simulink library "xrbsComm_r4"  (Simulink 7.1)
PreLoadFcn:
  | warning('off','MATLAB:mex:deprecatedExtension');xlmeta;com.xilinx.sysgen.util.StrategyUtil.loadAllStrategyNames();
undefined symbols (not defined in the file or in its folder): calc_path_data, gcbh, mfcm_matrix_rom, oct2dec, xlBlockLoadCallback
libraries: xbsIndex_r4 x851, mfcm_block_lib_v1 x5, xrbsComm_r4 x1, mfcm_misc_lib_v1 x1
(part 1 of 8)
settings Model: Tag=SysGenIndex  Creator=singhj  LastModifiedBy=sysgengroup

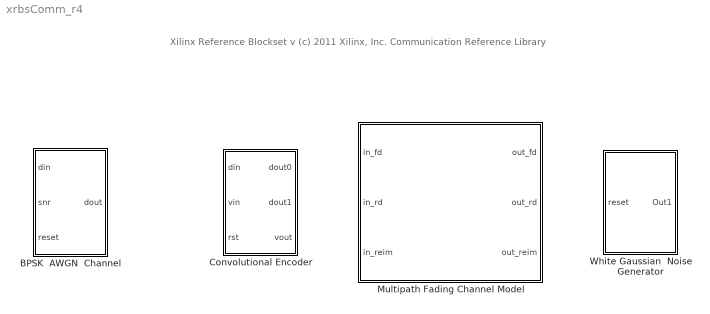
== system xrbsComm_r4 ==
  note: Xilinx Reference Blockset v
      | (c) 2011 Xilinx, Inc.
      |
      | Communication Reference Library
  BPSK  AWGN  Channel : Subsystem  mask(BPSK AWGN Channel){seed=510}
      mask prompts: seed "Decimal Seed Value"
      mask help: Binary Phase Shift Keying Additive White Gaussian Noise Channel. Adds scaled white Gaussian nose to an input signal.
      mask init:
      | [bg,fg] = xlcmap('XBlock',0);
      | iPos = get_param(gcb,'Position');
      | iWidth=iPos(3)-iPos(1); iHeight=iPos(4)-iPos(2);
      | iCx=iWidth/2;
      | iCy=iHeight/2;
      | [logoX, logoY] = xlogo(iPos);
      mask Help: eval('');xlDoc('-book','sysgen','-topic','BPSK_AWGN_Channel');
      mask Display:
      | patch([0 iWidth iWidth 0],[0 0 iHeight iHeight] , bg);
      | patch(logoX,logoY , fg);
      | port_label('input',1,'din');
      | port_label('input',2,'snr');
      | port_label('input',3,'reset');
      | port_label('output',1,'dout');
      | plot([0 0 iWidth iWidth 0], [0 iHeight iHeight 0 0]);
  Convolutional Encoder : Subsystem  mask(Convolutional Encoder Reference Block){K=7, code=[177 133]}
      mask prompts: K "Constraint Length [3 to 9]"; code "Convolutional code array (octal)"
      mask help: The constraint length and convolution code array are controlled by the mask parameters.
      mask init:
      | saved_gcb = gcb;
      | % Because of an issue where I was unable to save state consistently 
      | % when changing parameters and clicking the 'Apply' button, 
      | % I have included the following workaround that determines the number of subsystems.
      | sys_in_convenc = find_system(saved_gcb, 'lookUnderMasks', 'all', 'SearchDepth', 1, 'BlockType', 'SubSystem');
      | subsys_in_convenc = strfind(sys_in_convenc(1:length(sys_in_convenc)), 'Subsystem');
      | found_num_sys = 2;
      | for idx = 1:length(subsys_in_convenc)
      |   if (length(subsys_in_convenc(idx)))
      |     start_of_str = subsys_in_convenc{idx};
      |     length_of_sstr = length('Subsystem');
      |     char_idx_of_interest = start_of_str+length_of_sstr;
      |     
      |     if (char_idx_of_interest <= length(sys_in_convenc{idx}))
      |       char_of_interest = sys_in_convenc{idx}(char_idx_of_interest);
      |       sys_num = str2num(char_of_interest) + 1;
      |       if (sys_num > found_num_sys)
      |         found_num_sys = sys_num;
      |       end
      |     end
      |   end
      | end
      | saved_existing_subsys = found_num_sys;  
      | 
      | 
      | % Code for drawing the System Generator icon.
      | 
      | [bg,fg] = xlcmap('XBlock',0);
      | iPos = get_param(gcb,'Position');
      | iWidth=iPos(3)-iPos(1); iHeight=iPos(4)-iPos(2);
      | iCx=iWidth/2;
      | iCy=iHeight/2;
      | [logoX, logoY] = xlogo(iPos);
      | 
      | 
      | 
      | % Perform error checking on input parameters
      | 
      | err__k_not_int_in_range = false;
      | err__k_not_evaluated = false;
      | if (length(K) ~= 0)
      |   k_int = int32(round(K));
      |   if ((k_int ~= K) | (k_int < 3) | (k_int > 9))
      |     err__k_not_int_in_range = true;
      |   end
      | else
      |   err__k_not_evaluated = true;
      | end
      | err_in_param_k = err__k_not_int_in_range | err__k_not_evaluated;
      | 
      | err__codelen_not_in_range = false;
      | err__code_not_octal = false;
      | err__code_too_large_for_constraint = false;
      | err__code_not_evaluated = false;
      | if (length(code) ~= 0)
      |   code_len = length(code);
      |   if ((code_len < 2) | (code_len > 7))
      |     err__codelen_not_in_range = true;
      |   end
      |   for idx = 1:code_len
      |     try
      |       oct2dec(code(idx));
      |     catch
      |       err__code_not_octal = idx;
      |     end
      |   end
      |   if (~err_in_param_k & (err__code_not_octal == 0))
      |     code_eval_dec = oct2dec(code);
      |     max_code_val = 2^k_int;
      |     err__code_too_large_for_constraint = find(code_eval_dec > max_code_val);
      |     if (length(err__code_too_large_for_constraint) == 0)
      |       err__code_too_large_for_constraint = false;
      |     end
      |   end
      | else
      |   err__code_not_evaluated = true;
      | end
      | err_in_param_code = err__codelen_not_in_range | err__code_not_octal | err__code_too_large_for_constraint | err__code_not_evaluated;
      | 
      | valid_parameters = ~(err_in_param_k | err_in_param_code);
      | 
      | 
      | 
      | % Perform programatic generation of the convolutional encoder if the parameters are valid.
      | 
      | num_subsystems = saved_existing_subsys;
      | if (valid_parameters)
      |   num_subsystems = code_len;
      |   iconStr = '';
      |   if (num_subsystems ~= saved_existing_subsys)  
      |     subsys_proto = [saved_gcb '/Subsystem'];
      |     subsys_proto_dimensions = get_param(subsys_proto, 'Position');
      |     subsys_x = subsys_proto_dimensions(1);
      |     subsys_y = subsys_proto_dimensions(2);
      |     subsys_width = abs(subsys_proto_dimensions(3) - subsys_x);
      |     subsys_height = abs(subsys_proto_dimensions(4) - subsys_y);
      |     distance_between = 1.5*subsys_height;
      |     subsys_x2 = subsys_x+subsys_width;
      | 
      |     subsys_oport = [saved_gcb '/dout0'];
      |     subsys_oport_dimensions = get_param(subsys_oport, 'Position');
      |     subsys_oport_x = subsys_oport_dimensions(1);
      |     subsys_oport_y = subsys_oport_dimensions(2);
      |     subsys_oport_width = abs(subsys_oport_dimensions(3) - subsys_oport_x);
      |     subsys_oport_height = abs(subsys_oport_dimensions(4) - subsys_oport_y);
      |     subsys_oport_x2 = subsys_oport_x+subsys_oport_width;
      |     
      |     subsys_iport_din = 'din/1';
      |     subsys_iport_rst = 'rst/1';
      |     subsys_iport_vin = 'vin/1';
      | 
      |     minimum_subsystems = 2;
      |     if (num_subsystems  < saved_existing_subsys)
      |       for idx = (num_subsystems+1):saved_existing_subsys
      |         subsys_name = ['Subsystem' num2str(idx-1)];
      |         subsys_full_path = [saved_gcb '/' subsys_name];
      | 
      |         oport_name = ['dout' num2str(idx-1)];
      |         oport_full_path = [saved_gcb '/' oport_name];
      |         subsys_output_port = [subsys_name '/1'];
      |         oport_input_port = [oport_name '/1'];
      |         delete_line(saved_gcb, subsys_output_port, oport_input_port);
      |         delete_block(oport_full_path);
      |         
      |         subsys_din_port = [subsys_name '/1'];
      |         subsys_rst_port = [subsys_name '/2'];
      |         subsys_vin_port = [subsys_name '/3'];
      |         delete_line(saved_gcb, subsys_iport_din, subsys_din_port);
      |         delete_line(saved_gcb, subsys_iport_rst, subsys_rst_port);
      |         delete_line(saved_gcb, subsys_iport_vin, subsys_vin_port);
      |         delete_block(subsys_full_path);
      |       end
      |     elseif (num_subsystems > saved_existing_subsys)
      |       for idx = (saved_existing_subsys+1):num_subsystems
      |         subsys_name = ['Subsystem' num2str(idx-1)];
      |         new_subsys = [saved_gcb '/' subsys_name];
      |         y1 = subsys_y+(idx-1)*distance_between;
      |         y2 = subsys_y+subsys_height+(idx-1)*distance_between;
      |         new_position = [subsys_x y1 subsys_x2 y2];
      |         add_block(subsys_proto, new_subsys, 'Position', new_position);
      |         set_param(new_subsys, 'index', num2str(idx));
      |         
      |         oport_name = ['dout' num2str(idx-1)];
      |         new_oport = [saved_gcb '/' oport_name];
      |         y1 = subsys_oport_y+(idx-1)*distance_between;
      |         y2 = subsys_oport_y+subsys_oport_height+(idx-1)*distance_between;
      |         new_position = [subsys_oport_x y1 subsys_oport_x2 y2];
      |         add_block(subsys_oport, new_oport, 'Position', new_position);
      |         
      |         subsys_output_port = [subsys_name '/1'];
      |         oport_input_port = [oport_name '/1'];
      |         add_line(saved_gcb, subsys_output_port, oport_input_port);
      |         
      |         subsys_din_port = [subsys_name '/1'];
      |         subsys_rst_port = [subsys_name '/2'];
      |         subsys_vin_port = [subsys_name '/3'];
      |         add_line(saved_gcb, subsys_iport_din, subsys_din_port, 'autorouting', 'on');
      |         add_line(saved_gcb, subsys_iport_rst, subsys_rst_port, 'autorouting', 'on');
      |         add_line(saved_gcb, subsys_iport_vin, subsys_vin_port, 'autorouting', 'on');
      |       end
      |     end
      |       
      |     % Delete/Re-add the vout block to get the port numbers so that all dout ports
      |     % are grouped together.
      |     vout_block = [saved_gcb '/vout'];
      |     vout_block_pos = get_param(vout_block, 'Position');
      |     delete_block(vout_block);
      |     add_block(subsys_oport, vout_block, 'Position', vout_block_pos);
      |   end
      | else
      |   iconStr = 'ERROR';
      | end
      | 
      | 
      | 
      | % This code generates a vector and cellarray of
      | % port numbers and names respectively to allow
      | % the number of output ports to be changed.
      | % (Their is no way to change the icon Drawing
      | % Code dynamically--i.e. it doesn't allow
      | % loop constructs, hence all the add ports.)
      | 
      | num_dout_ports = num_subsystems;
      | max_out_ports = 8;
      | out_port_nums = [];
      | out_port_names = {};
      | for idx = 1:max_out_ports
      |   if (idx <= num_dout_ports)
      |     out_port_nums = [out_port_nums idx];
      |     out_port_names = [out_port_names {['dout' num2str(idx)]}];
      |   else
      |     out_port_nums = [out_port_nums (num_dout_ports+1)];
      |     out_port_names = [out_port_names {'vout'}];
      |   end;
      | end
      | 
      | 
      | 
      | % Present any errors or warnings to users
      | 
      | if (err__k_not_evaluated)
      |   errordlg([saved_gcb ': Constraint length could not be evaluated.']);
      | elseif (err__k_not_int_in_range)
      |   errordlg([saved_gcb ': Constraint length is set to ' num2str(K) ', but must be an integer between 3 and 9, inclusive.']);
      | elseif(err__code_not_evaluated)
      |   errordlg([saved_gcb ': The convolution code array could not be evaluated.']);
      | elseif(err__code_too_large_for_constraint)
      |   errordlg([saved_gcb ': The convolution code array value(s) at position(s): ' num2str(err__code_too_large_for_constraint) ', are too large for the constraint length, ' num2str(K) '.']);
      | elseif(err__code_not_octal)
      |   errordlg([saved_gcb ': The convolution code array must contain octal numbers only (i.e. only numbers containing the digits 0-7).  The value at position ' num2str(err__code_not_octal) ' is not an octal value.']);
      | elseif(err__codelen_not_in_range)
      |   errordlg([saved_gcb ': The length of the convolution code array must be between 2 and 7, inclusive.']);
      | end
      settings: CopyFcn=set_param(gcb, 'MaskSelfModifiable', 'on', 'LinkStatus', 'none');
      mask Help: eval('');xlDoc('-book','sysgen','-topic','Convolutional_Encoder');
      mask Display:
      | patch([0 iWidth iWidth 0],[0 0 iHeight iHeight] , bg);
      | patch(logoX,logoY , fg);
      | port_label('input',1,'din');
      | port_label('input',2,'vin');
      | port_label('input',3,'rst');
      | port_label('output', out_port_nums(1), char(out_port_names{1}));
      | port_label('output', out_port_nums(2), char(out_port_names{2}));
      | port_label('output', out_port_nums(3), char(out_port_names{3}));
      | port_label('output', out_port_nums(4), char(out_port_names{4}));
      | port_label('output', out_port_nums(5), char(out_port_names{5}));
      | port_label('output', out_port_nums(6), char(out_port_names{6}));
      | port_label('output', out_port_nums(7), char(out_port_names{7}));
      | port_label('output', out_port_nums(8), char(out_port_names{8}));
      | disp(iconStr, 'texmode', 'on');
      | plot([0 0 iWidth iWidth 0], [0 iHeight iHeight 0 0]);
  Multipath Fading Channel Model : Subsystem  LoadFcn=xlBlockLoadCallback(gcbh);  mask(Multipath Fading Channel Model Block){infoedit=Multipath Fading Channel Model., DELAY=[0], GAIN=[1], RT=eye(4,4), RR=eye(4,4), SPEC_DATA=calc_path_data(zeros(4,4,1)+2,ones(4,4,1)), RATE=64, DATAPATH_WIDTH=18, TX_BINPT=17, FADE_BINPT=15, RX_BINPT=15, MAT_BINPT=17, SEED='461AF8228C9F8C92', has_advanced_control=0, sggui_pos=-1,-1,-1,-1, block_type=mfcm, block_version=, sg_icon_stat=180,156,-1,-1,white,blue,0,07734,right,,[ ],[ ], sg_mask_display=|, sg_list_contents=, sg_blockgui_xml=}
      mask sg_mask_display=|
      | fprintf('','COMMENT: begin icon graphics');
      | patch([0 180 180 0 0 ],[0 0 156 156 0 ],[0.77 0.82 0.91 ]);
      | plot([0 180 180 0 0 ],[0 0 156 156 0 ]);
      | patch([41.05 72.84 94.84 116.84 138.84 94.84 63.05 41.05 ],[102.42 102.42 124.42 102.42 124.42 124.42 124.42 102.42 ],[1 1 1 ]);
      | patch([63.05 94.84 72.84 41.05 63.05 ],[80.42 80.42 102.42 102.42 80.42 ],[0.931 0.946 0.973 ]);
      | patch([41.05 72.84 94.84 63.05 41.05 ],[58.42 58.42 80.42 80.42 58.42 ],[1 1 1 ]);
      | patch([63.05 138.84 116.84 94.84 72.84 41.05 63.05 ],[36.42 36.42 58.42 36.42 58.42 58.42 36.42 ],[0.931 0.946 0.973 ]);
      | fprintf('','COMMENT: end icon graphics');
      | fprintf('','COMMENT: begin icon text');
      | fprintf('','COMMENT: end icon text');disp(sprintf('Tx=%d Rx=%d\nPATHS=%d',size(RT,1),size(RR,1),length(GAIN)),'texmode','on');
      mask prompts: infoedit ""; DELAY "Path Delay Vector"; GAIN "Path Gain Vector"; RT "Transmit Array Spatial Covariance Matrices"; RR "Receive Array Spatial Covariance Matrices"; SPEC_DATA "Spectrum Data"; DATAPATH_WIDTH "Datapath Width in Bits"; TX_BINPT "Transmit Multiply Binary Point"; FADE_BINPT "Fading Multiply Binary Point"; RX_BINPT "Receive Multiply Binary Point"; MAT_BINPT "Covariance Matrix Binary Point"; SEED "Random Seed"; has_advanced_control ""; sggui_pos ""; block_type ""; block_version ""; sg_icon_stat ""; sg_mask_display ""; sg_list_contents ""; sg_blockgui_xml ""
      mask help: Multipath Fading Channel Model.
      mask init:
      | try
      |   tmp_gcb = gcb;
      |   tmp_gcbh = gcbh;
      |   if (strcmp('SysGenIndex',get_param(bdroot(tmp_gcbh),'tag')) && ~isempty(regexp(bdroot(tmp_gcb), '^xbs', 'once')))
      |     return;
      |   end;
      |   xlMungeMaskParams;
      | 
      |   block_type='mfcm';
      | 
      |   serialized_declarations = '{''block_type''=>''String''}';
      |   ptable_ = xlblockprep(get_param(tmp_gcb, 'MaskWSVariables'));
      |   try
      |     xlBlockMoveCallback(tmp_gcbh);
      |   catch 
      |      clear global xl_updateicon_recursion_guard;
      |   end;
      | catch
      |   global dbgsysgen;
      |   if(~isempty(dbgsysgen) && dbgsysgen)
      |     e = regexprep(lasterr, '\n', '\nError: ');
      |     disp(['Error: While running MaskInit code on block ' tmp_gcb ': ' e]);
      |     error(e);
      |   end
      | end
      settings: CopyFcn=xlBlockMoveCallback(gcbh);  DeleteFcn=xlDestroyGui(gcbh);  ModelCloseFcn=xlDestroyGui(gcbh);  PreSaveFcn=xlBlockPreSaveCallback(gcbh);  PostSaveFcn=xlBlockPostSaveCallback(gcbh);  DestroyFcn=xlDestroyGui(gcbh);  OpenFcn=xlOpenGui(gcbh, 'mfcm_gui.xml', -1, -1)  CloseFcn=xlDestroyGui(gcbh);  MoveFcn=xlBlockMoveCallback(gcbh);
      mask Help: eval('');xlDoc('-book','sysgen','-topic','Multipath_Fading_Channel_Model');
      mask Display:
      | fprintf('','COMMENT: begin icon graphics');
      | patch([0 180 180 0 0 ],[0 0 156 156 0 ],[0.77 0.82 0.91 ]);
      | plot([0 180 180 0 0 ],[0 0 156 156 0 ]);
      | patch([41.05 72.84 94.84 116.84 138.84 94.84 63.05 41.05 ],[102.42 102.42 124.42 102.42 124.42 124.42 124.42 102.42 ],[1 1 1 ]);
      | patch([63.05 94.84 72.84 41.05 63.05 ],[80.42 80.42 102.42 102.42 80.42 ],[0.931 0.946 0.973 ]);
      | patch([41.05 72.84 94.84 63.05 41.05 ],[58.42 58.42 80.42 80.42 58.42 ],[1 1 1 ]);
      | patch([63.05 138.84 116.84 94.84 72.84 41.05 63.05 ],[36.42 36.42 58.42 36.42 58.42 58.42 36.42 ],[0.931 0.946 0.973 ]);
      | fprintf('','COMMENT: end icon graphics');
      | fprintf('','COMMENT: begin icon text');
      | fprintf('','COMMENT: end icon text');disp(sprintf('Tx=%d Rx=%d\nPATHS=%d',size(RT,1),size(RR,1),length(GAIN)),'texmode','on');
  White Gaussian  Noise Generator : Subsystem  mask(White Gaussian Noise Generator){seed=512}
      mask help: White Gaussian Noise Generator. Generates white Gaussian noise using a combination of the Box-Muller algorithm and the central limit theorem.
      mask init:
      | old_seed = rand('seed');
      | rand('seed',seed);
      | init1 = [dec2hex(floor(rand*16)) dec2hex(floor(rand*16)) dec2hex(floor(rand*16)) ...
      | 		dec2hex(floor(rand*16)) dec2hex(floor(rand*16)) dec2hex(floor(rand*16)) ...
      | 		dec2hex(floor(rand*16)) dec2hex(floor(rand*16)) dec2hex(floor(rand*16)) ...
      | 		dec2hex(floor(rand*16)) dec2hex(floor(rand*16)) dec2hex(floor(rand*16))];
      | seed1 = hex2dec(init1);
      | init2 = [dec2hex(floor(rand*16)) dec2hex(floor(rand*16)) dec2hex(floor(rand*16)) ...
      | 		dec2hex(floor(rand*16)) dec2hex(floor(rand*16)) dec2hex(floor(rand*16)) ...
      | 		dec2hex(floor(rand*16)) dec2hex(floor(rand*16)) dec2hex(floor(rand*16)) ...
      | 		dec2hex(floor(rand*16)) dec2hex(floor(rand*16)) dec2hex(floor(rand*16))];
      | seed2 = hex2dec(init2);
      | init3 = [dec2hex(floor(rand*16)) dec2hex(floor(rand*16)) dec2hex(floor(rand*16)) ...
      | 		dec2hex(floor(rand*16)) dec2hex(floor(rand*16)) dec2hex(floor(rand*16)) ...
      | 		dec2hex(floor(rand*16)) dec2hex(floor(rand*16)) dec2hex(floor(rand*16)) ...
      | 		dec2hex(floor(rand*16)) dec2hex(floor(rand*16)) dec2hex(floor(rand*16))];
      | seed3 = hex2dec(init3);
      | init4 = [dec2hex(floor(rand*16)) dec2hex(floor(rand*16)) dec2hex(floor(rand*16)) ...
      | 		dec2hex(floor(rand*16)) dec2hex(floor(rand*16)) dec2hex(floor(rand*16)) ...
      | 		dec2hex(floor(rand*16)) dec2hex(floor(rand*16)) dec2hex(floor(rand*16)) ...
      | 		dec2hex(floor(rand*16)) dec2hex(floor(rand*16)) dec2hex(floor(rand*16))];
      | seed4 = hex2dec(init4);
      | rand('seed',old_seed);
      | 
      | 
      | [bg,fg] = xlcmap('XBlock',0);
      | iPos = get_param(gcb,'Position');
      | iWidth=iPos(3)-iPos(1); iHeight=iPos(4)-iPos(2);
      | iCx=iWidth/2;
      | iCy=iHeight/2;
      | [logoX, logoY] = xlogo(iPos);
      mask Help: eval('');xlDoc('-book','sysgen','-topic','White_Gaussian_Noise_Generator');
      mask Display:
      | patch([0 iWidth iWidth 0],[0 0 iHeight iHeight] , bg);
      | patch(logoX,logoY , fg);
      | port_label('input',1,'reset');
      | port_label('output',1,'noise');
      | plot([0 0 iWidth iWidth 0], [0 iHeight iHeight 0 0]);

== system xrbsComm_r4/BPSK  AWGN  Channel ==
  note: The WGNG block generates a probability density function (PDF) that is Gaussian to within .2% for
      | 4.8 standard deviations from the mean.  The PDF is scaled based on the value of the signal to noise
      | ratio to achieve the desired noise variance.  The SNR input is defined as (Eb/No) in dB for uncoded BPSK
      | with unit symbol energy (Es = 1).  If the SNR input is of type UFix8_4, the valid range is from 0.0 to 15.9375
      | in steps of 0.0625dB.  To use the AWGN in a system with coding and/or to use the core with different
      | modulation formats, it is necessary to adjust the SNR value to accommodate the difference in spectral
      | efficiency.  If we have BPSK modulation with rate 1/2 coding and keep Es = 1and No constant, then Eb = 2
      | and Eb/No = SNR + 3 dB.  If we have uncoded QPSK modulation with I = +/-1 and Q = +/-1 and add
      | independent noise sequences, then each channel looks like and independent BPSK channel and the
      | Eb/No = SNR.  If we then add rate 1/2 coding to the QPSK case, we have Eb/No = SNR + 3 dB.
      |
      | For more information see:
      |
      | [1] A. Ghazel, E. Boutillon, J. L. Danger, G. Gulak and H. Laamari, "Design and Performance Analysis of a
      | High Speed AWGN Communication Channel Emulator" IEEE PACRIM Conference, Victoria, B. C., Aug.
      | 2001.
      | [2] Xilinx Data Sheet: Additive White Gaussian Noise (AWGN) Core v1.0, Xilinx, Inc. October 2002
  din : Inport  OutDataType=sfix(16)  OutScaling=2^0
  snr : Inport  Port=2  OutDataType=sfix(16)  OutScaling=2^0
  reset : Inport  Port=3  OutDataType=sfix(16)  OutScaling=2^0
  AddSub : xbsIndex_r4/AddSub  mode=Addition  use_carryin=off  use_carryout=off  en=off  latency=1  precision=Full  arith_type=Unsigned  n_bits=8  bin_pt=2  quantization=Truncate  overflow=Wrap  dbl_ovrd=off  use_behavioral_HDL=on  pipelined=off  use_rpm=off  block_type=addsub
      settings: xl_area=[0, 0, 0, 0, 0, 0, 0]  block_version=VER_STRING_GOES_HERE
  Constant1 : xbsIndex_r4/Constant  arith_type=Signed (2's comp)  const=1  n_bits=2  bin_pt=0  explicit_period=off  period=1  equ=P=C  opselect=C  inp2=PCIN>>17  opr=+  inp1=P  carry=CIN  dbl_ovrd=off  block_type=constant
      settings: block_version=VER_STRING_GOES_HERE
  Constant2 : xbsIndex_r4/Constant  arith_type=Signed (2's comp)  const=-1  n_bits=2  bin_pt=0  explicit_period=off  period=1  equ=P=C  opselect=C  inp2=PCIN>>17  opr=+  inp1=P  carry=CIN  dbl_ovrd=off  block_type=constant
      settings: block_version=VER_STRING_GOES_HERE
  Convert : xbsIndex_r4/Convert  arith_type="Signed  (2's comp)"  n_bits=16  bin_pt=11  quantization="Round  (unbiased: +/- Inf)"  overflow=Wrap  latency=2  dbl_ovrd=off  pipeline=off  block_type=convert
      settings: infoedit=The input is presented at the output after quantization and overflow effects.<P><P>Hardware notes: Additional hardware is used when rounding or saturation is selected and output width is less than the input width.  xl_area=[0, 0, 0, 0, 0, 0, 0]  block_version=VER_STRING_GOES_HERE
  Delay : xbsIndex_r4/Delay  en=off  latency=14  dbl_ovrd=off  reg_retiming=off  block_type=delay
      settings: infoedit="Delay line having  configurable length.<P><P>Hardware notes: A delay line is a chain, each link of which is an SRL16 followed by a flip-flop. If register retiming is enabled, the delay line is a chain of flip-flops."  xl_area=[0, 0, 0, 0, 0, 0, 0]  block_version=VER_STRING_GOES_HERE
  Input  Conversion : Subsystem
  Mult : xbsIndex_r4/Mult  precision=Full  arith_type="Signed  (2's comp)"  n_bits=8  bin_pt=2  quantization=Truncate  overflow=Wrap  en=off  latency=2  dbl_ovrd=off  use_behavioral_HDL=off  use_embedded=on  pipeline=off  use_rpm=off  placement_style=Rectangular shape  block_type=mult
      settings: infoedit=Multiplies two values.<P><P>Hardware notes: To use the internal pipeline stage of the dedicated multiplier you must select 'Pipeline to Greatest Extent Possible'.  xl_area=[0, 0, 0, 0, 0, 0, 0]  block_version=VER_STRING_GOES_HERE
  Mux : xbsIndex_r4/Mux  inputs=2  en=off  latency=0  precision=Full  arith_type="Signed  (2's comp)"  n_bits=8  bin_pt=2  quantization=Truncate  overflow=Wrap  dbl_ovrd=off  block_type=mux
      settings: xl_area=[0, 0, 0, 0, 0, 0, 0]  block_version=VER_STRING_GOES_HERE
  ROM : xbsIndex_r4/ROM  depth=256  initVector=((2*10.^(0.1*(([0:255]/10) - 0.6*floor([0:255]/16) ))).^(-0.5))*1.0023  distributed_mem=Block RAM  rst=off  init_reg=0  en=off  latency=1  arith_type=Unsigned  n_bits=15  bin_pt=15  dbl_ovrd=off  use_rpm=off  block_type=sprom
      settings: xl_area=[0, 0, 0, 0, 0, 0, 0]  block_version=VER_STRING_GOES_HERE
  White Gaussian  Noise Generator : xrbsComm_r4/White Gaussian  Noise Generator  seed=seed
  dout : Outport  OutDataType=sfix(16)  OutScaling=2^0
  wires:
  reset/1 -> White Gaussian  Noise Generator/1
  Delay/1 -> AddSub/1
  Convert/1 -> AddSub/2
  White Gaussian  Noise Generator/1 -> Mult/2
  din/1 -> Mux/1
  snr/1 -> Input  Conversion/1(" ")
  Mult/1 -> Convert/1
  ROM/1 -> Mult/1
  AddSub/1 -> dout/1
  Input  Conversion/1(conv) -> ROM/1
  Constant1/1 -> Mux/2
  Constant2/1 -> Mux/3
  Mux/1 -> Delay/1

== system xrbsComm_r4/Convolutional Encoder ==
  din : Inport  OutDataType=sfix(16)  OutScaling=2^0
  vin : Inport  Port=2  OutDataType=sfix(16)  OutScaling=2^0
  rst : Inport  Port=3  OutDataType=sfix(16)  OutScaling=2^0
  More Info : Subsystem
      mask Display: disp('Double click\n for\n more information.')
  Subsystem : Subsystem  mask{index=1}
  Subsystem1 : Subsystem  mask{index=2}
  Valid Out Logic : Subsystem
  dout0 : Outport  OutDataType=sfix(16)  OutScaling=2^0
  dout1 : Outport  Port=2  OutDataType=sfix(16)  OutScaling=2^0
  vout : Outport  Port=3  OutDataType=sfix(16)  OutScaling=2^0
  wires:
  rst/1 -> Valid Out Logic/2(rst), Subsystem/2(rst), Subsystem1/2(rst)
  din/1 -> Subsystem1/1(din), Subsystem/1(din)
  Valid Out Logic/1(vout) -> vout/1
  Subsystem/1(dout) -> dout0/1
  Subsystem1/1(dout) -> dout1/1
  vin/1 -> Valid Out Logic/1(vin), Subsystem1/3(vin), Subsystem/3(vin)

== system xrbsComm_r4/Multipath Fading Channel Model ==
  in_fd : Inport  OutDataType=sfix(16)  OutScaling=2^0
  in_rd : Inport  Port=2  OutDataType=sfix(16)  OutScaling=2^0
  in_reim : Inport  Port=3  OutDataType=sfix(16)  OutScaling=2^0
  assert[in_fd] : mfcm_misc_lib_v1/assert_width_period  SystemSampleTime=-1  MIN_WIDTH=1  MAX_WIDTH=1  MIN_PERIOD=2*length(GAIN)*max(max(size(RT,1),size(RR,1))^2,size(RT,1)*size(RR,1)*ceil(64/RATE))  MAX_PERIOD=0
  input delay line : mfcm_block_lib_v1/input delay line  SystemSampleTime=-1  MT=size(RT,1)  DELAY=DELAY
  matrix ops : Subsystem  AncestorBlock=mfcm_lib_v1/Multipath Fading Channel Model/matrix ops  mask{MATS=mfcm_matrix_rom(RT,GAIN,RR)}
      mask prompts: MATS "Matrix ROM data"
  out_fd : Outport  OutDataType=sfix(16)  OutScaling=2^0
  out_rd : Outport  Port=2  OutDataType=sfix(16)  OutScaling=2^0
  out_reim : Outport  Port=3  OutDataType=sfix(16)  OutScaling=2^0
  wires:
  matrix ops/3(out_reim) -> out_reim/1
  matrix ops/2(out_rd) -> out_rd/1
  matrix ops/1(out_fd) -> out_fd/1
  in_reim/1 -> input delay line/3
  in_rd/1 -> input delay line/2
  in_fd/1 -> assert[in_fd]/1, input delay line/1
  input delay line/3 -> matrix ops/3(in_reim)
  input delay line/2 -> matrix ops/2(in_rd)
  input delay line/1 -> matrix ops/1(in_fd)

== system xrbsComm_r4/White Gaussian  Noise Generator ==
  note: The WGNG generates white Gaussian noise using a combination of the Box-Muller algorithm and the Central Limit Theorem
      | following the general approach described in [1].   The Box-Muller algorithm generates a unit normal random variable via a
      | transformation of two independent random variables that are uniformly distributed over [0,1].  This is accomplished by storing
      | Box-Muller function values in ROMs and addressing them with uniform random variables.  The uniform random variables are
      | produced by multiple-bit leap-forward LFSRs.  A standard LFSR generates one output per clock cycle.  K-bit leap-forward LFSRs
      | are able to generate k outputs in a single cycle.  For example, a 4-bit leap-forward LFSR outputs a discrete uniform random
      | variable between 0 and 15.  A portion of the 48-bit block parameter seed initializes each LFSR allowing customization.  The
      | outputs of four parallel Box-Muller subsystems are averaged to obtain a probability density function (PDF) that is Gaussian.
      | The overall latency of the WGNG is 10 clock cycles.  The output port noise is a 12 bit signed number with 7 bits after the binary
      | point.
      |
      | [1] A. Ghazel, E. Boutillon, J. L. Danger, G. Gulak and H. Laamari, "Design and Performance Analysis of a
      | High Speed AWGN Communication Channel Emulator" IEEE PACRIM Conference, Victoria, B. C., Aug. 2001.
  " reset" : Inport  OutDataType=sfix(16)  OutScaling=2^0
  AddSub : xbsIndex_r4/AddSub  mode=Addition  use_carryin=off  use_carryout=off  en=off  latency=1  precision=Full  arith_type=Unsigned  n_bits=8  bin_pt=2  quantization=Truncate  overflow=Wrap  dbl_ovrd=off  use_behavioral_HDL=on  pipelined=off  use_rpm=off  block_type=addsub
      settings: xl_area=[0, 0, 0, 0, 0, 0, 0]  block_version=VER_STRING_GOES_HERE
  AddSub1 : xbsIndex_r4/AddSub  mode=Addition  use_carryin=off  use_carryout=off  en=off  latency=1  precision=Full  arith_type=Unsigned  n_bits=8  bin_pt=2  quantization=Truncate  overflow=Wrap  dbl_ovrd=off  use_behavioral_HDL=on  pipelined=off  use_rpm=off  block_type=addsub
      settings: xl_area=[0, 0, 0, 0, 0, 0, 0]  block_version=VER_STRING_GOES_HERE
  AddSub2 : xbsIndex_r4/AddSub  mode=Addition  use_carryin=off  use_carryout=off  en=off  latency=1  precision=Full  arith_type=Unsigned  n_bits=8  bin_pt=2  quantization=Truncate  overflow=Wrap  dbl_ovrd=off  use_behavioral_HDL=on  pipelined=off  use_rpm=off  block_type=addsub
      settings: xl_area=[0, 0, 0, 0, 0, 0, 0]  block_version=VER_STRING_GOES_HERE
  Box-Muller1 : Subsystem  mask(Box-Muller){f_init1=bitget(seed1, 17:-1:1), f_init2=bitget(seed1, 25:-1:1), f_init3=bitget(seed1, 29:-1:1), f_init4=bitget(seed1, 31:-1:1), f_init5=bitget(seed1, 41:-1:1), g_init=bitget(seed1, 47:-1:1)}
      mask prompts: f_init1 "f_init1(17:1)"; f_init2 "f_init2(25:1)"; f_init3 "f_init3(29:1)"; f_init4 "f_init4(31:1)"; f_init5 "f_init5(41:1)"; g_init "g_init(47:1)"
  Box-Muller2 : Subsystem  mask(Box-Muller){f_init1=bitget(seed2, 17:-1:1), f_init2=bitget(seed2, 25:-1:1), f_init3=bitget(seed2, 29:-1:1), f_init4=bitget(seed2, 31:-1:1), f_init5=bitget(seed2, 41:-1:1), g_init=bitget(seed2, 47:-1:1)}
      mask prompts: f_init1 "f_init1(17:1)"; f_init2 "f_init2(25:1)"; f_init3 "f_init3(29:1)"; f_init4 "f_init4(31:1)"; f_init5 "f_init5(41:1)"; g_init "g_init(47:1)"
  Box-Muller3 : Subsystem  mask(Box-Muller){f_init1=bitget(seed3, 17:-1:1), f_init2=bitget(seed3, 25:-1:1), f_init3=bitget(seed3, 29:-1:1), f_init4=bitget(seed3, 31:-1:1), f_init5=bitget(seed3, 41:-1:1), g_init=bitget(seed3,47:-1:1)}
      mask prompts: f_init1 "f_init1(17:1)"; f_init2 "f_init2(25:1)"; f_init3 "f_init3(29:1)"; f_init4 "f_init4(31:1)"; f_init5 "f_init5(41:1)"; g_init "g_init(47:1)"
  Box-Muller4 : Subsystem  mask(Box-Muller){f_init1=bitget(seed4, 17:-1:1), f_init2=bitget(seed4, 25:-1:1), f_init3=bitget(seed4, 29:-1:1), f_init4=bitget(seed4, 31:-1:1), f_init5=bitget(seed4, 41:-1:1), g_init=bitget(seed4, 47:-1:1)}
      mask prompts: f_init1 "f_init1(17:1)"; f_init2 "f_init2(25:1)"; f_init3 "f_init3(29:1)"; f_init4 "f_init4(31:1)"; f_init5 "f_init5(41:1)"; g_init "g_init(47:1)"
  Reinterpret : xbsIndex_r4/Reinterpret  force_arith_type=off  arith_type=Unsigned  force_bin_pt=on  bin_pt=7  block_type=cast
      settings: infoedit="Changes type of samples without altering their binary representation.<P><P>Hardware notes: In hardware this block costs nothing.<P><P>Example:  Suppose the input is 6 bits wide, signed, with 2 fractional bits, and the output is forced to unsigned with 0 fractional bits.  Then an input of -2.0 (1110.00 in binary 2's complement) becomes an output of 56 (111000 in binary)."  block_version=VER_STRING_GOES_HERE
  Out1 : Outport  OutDataType=sfix(16)  OutScaling=2^0
  wires:
  " reset"/1 -> Box-Muller3/1(reset), Box-Muller4/1(reset), Box-Muller2/1(reset), Box-Muller1/1(" reset")
  Reinterpret/1 -> Out1/1
  Box-Muller4/1(bm) -> AddSub1/2
  Box-Muller3/1(bm) -> AddSub1/1
  Box-Muller2/1(bm) -> AddSub/2
  Box-Muller1/1(bm) -> AddSub/1
  AddSub2/1 -> Reinterpret/1
  AddSub1/1 -> AddSub2/2
  AddSub/1 -> AddSub2/1

== system xrbsComm_r4/BPSK  AWGN  Channel/Input  Conversion ==
  " " : Inport  OutDataType=sfix(16)  OutScaling=2^0
  AddSub1 : xbsIndex_r4/AddSub  mode=Addition  use_carryin=off  use_carryout=off  en=off  latency=0  precision=User Defined  arith_type=Unsigned  n_bits=8  bin_pt=0  quantization=Truncate  overflow=Wrap  dbl_ovrd=off  use_behavioral_HDL=on  pipelined=off  use_rpm=off  block_type=addsub
      settings: xl_area=[0, 0, 0, 0, 0, 0, 0]  block_version=VER_STRING_GOES_HERE
  CMult : xbsIndex_r4/CMult  const=16  const_n_bits=5  const_bin_pt=0  en=off  latency=0  precision=Full  arith_type="Signed  (2's comp)"  n_bits=8  bin_pt=6  quantization="Round  (unbiased: +/- Inf)"  overflow=Wrap  dbl_ovrd=off  use_behavioral_HDL=off  mem_type=Distributed RAM  placement_style=Rectangular Shape  pipeline=off  use_rpm=off  block_type=cmult
      settings: xl_area=[0, 0, 0, 0, 0, 0, 0]  block_version=VER_STRING_GOES_HERE
  CMult1 : xbsIndex_r4/CMult  const=10  const_n_bits=4  const_bin_pt=0  en=off  latency=0  precision=Full  arith_type="Signed  (2's comp)"  n_bits=8  bin_pt=6  quantization="Round  (unbiased: +/- Inf)"  overflow=Wrap  dbl_ovrd=off  use_behavioral_HDL=off  mem_type=Distributed RAM  placement_style=Rectangular Shape  pipeline=off  use_rpm=off  block_type=cmult
      settings: xl_area=[0, 0, 0, 0, 0, 0, 0]  block_version=VER_STRING_GOES_HERE
  Shift : xbsIndex_r4/Shift  shift_dir=Right  shift_bits=4  en=off  latency=0  precision=User Defined  arith_type=Unsigned  n_bits=4  bin_pt=0  quantization=Truncate  overflow=Wrap  dbl_ovrd=off  block_type=shift
      settings: xl_area=[0, 0, 0, 0, 0, 0, 0]  block_version=VER_STRING_GOES_HERE
  Slice : xbsIndex_r4/Slice  nbits=4  boolean_output=off  mode=Upper Bit Location + Width  bit1=0  base1=MSB of Input  bit0=0  base0=LSB of Input  dbl_ovrd=off  block_type=slice
      settings: infoedit="Extracts a given range of bits from each input sample and presents it at the output.  The output type is ordinarily unsigned with binary point at zero, but can be Boolean when the slice is one bit wide.<P><P>Hardware notes: In hardware this block costs nothing."  block_version=VER_STRING_GOES_HERE
  Slice1 : xbsIndex_r4/Slice  nbits=4  boolean_output=off  mode=Lower Bit Location + Width  bit1=0  base1=MSB of Input  bit0=0  base0=LSB of Input  dbl_ovrd=off  block_type=slice
      settings: infoedit="Extracts a given range of bits from each input sample and presents it at the output.  The output type is ordinarily unsigned with binary point at zero, but can be Boolean when the slice is one bit wide.<P><P>Hardware notes: In hardware this block costs nothing."  block_version=VER_STRING_GOES_HERE
  conv : Outport  OutDataType=sfix(16)  OutScaling=2^0
  wires:
  Slice/1 -> CMult/1
  Slice1/1 -> CMult1/1
  AddSub1/1 -> conv/1
  CMult/1 -> AddSub1/1
  " "/1 -> Slice/1, Slice1/1
  CMult1/1 -> Shift/1
  Shift/1 -> AddSub1/2

== system xrbsComm_r4/Convolutional Encoder/More Info ==
  note: For example, the octal convolutional codes
      | are shifted and bits from those are used to
      | drive the inputs of the AND gates at left.
      | Any AND gate with a '1' on one input will
      | collapse to a wire.  Any AND gate with a '0'
      | on one input will get pruned away, along
      | with all logic driving the other input of the
      | AND gate.
  note: When the AND gates get pruned, some of the
      | XOR gates have a constant 0 input.  These
      | will get pruned as well.
  note: The 9-bit shift register has been replicated twice
      | simply to make the drawing cleaner.  The
      | synthesizer will collapse these three registers
      | into a single 9-bit shifter.
  note: This block works using a form of parameterizable
      | mux-based collapsing.  This is a method in which
      | constants drive logic blocks.  All logic driven by
      | a constant will be optimized away by the
      | sythesizer.
  note: Parameterizable Mux-Based Collapsing

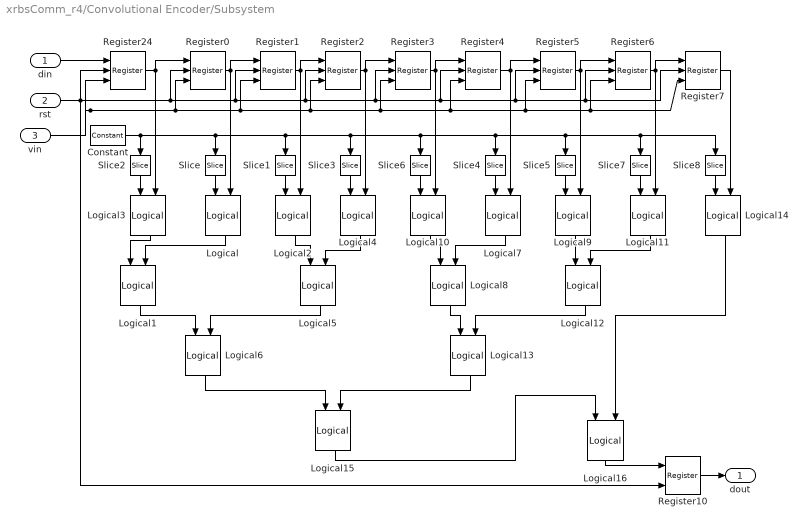
== system xrbsComm_r4/Convolutional Encoder/Subsystem ==
  din : Inport  OutDataType=sfix(16)  OutScaling=2^0
  rst : Inport  Port=2  OutDataType=sfix(16)  OutScaling=2^0
  vin : Inport  Port=3  OutDataType=sfix(16)  OutScaling=2^0
  Constant : xbsIndex_r4/Constant  arith_type=Unsigned  const=oct2dec(code(index))*2^(9-K)  n_bits=9  bin_pt=0  explicit_period=off  period=1  equ=P=C  opselect=C  inp2=PCIN>>17  opr=+  inp1=P  carry=CIN  dbl_ovrd=off  block_type=constant
      settings: block_version=VER_STRING_GOES_HERE
  Logical{,2..4,7,9..11,14} (9 alike) : xbsIndex_r4/Logical  Orientation=down  logical_function=AND  inputs=2  en=off  latency=0  precision=Full  arith_type=Unsigned  n_bits=16  bin_pt=0  align_bp=on  dbl_ovrd=off  block_type=logical
      settings: block_version=VER_STRING_GOES_HERE
  Logical{1,5..6,8,12..13,15..16} (8 alike) : xbsIndex_r4/Logical  Orientation=down  logical_function=XOR  inputs=2  en=off  latency=0  precision=Full  arith_type=Unsigned  n_bits=16  bin_pt=0  align_bp=on  dbl_ovrd=off  block_type=logical
      settings: block_version=VER_STRING_GOES_HERE
  Register{0..7,24} (9 alike) : xbsIndex_r4/Register  init=0  rst=on  en=on  dbl_ovrd=off  block_type=register
      settings: block_version=VER_STRING_GOES_HERE
  Register10 : xbsIndex_r4/Register  init=0  rst=on  en=off  dbl_ovrd=off  block_type=register
      settings: block_version=VER_STRING_GOES_HERE
  Slice : xbsIndex_r4/Slice  Orientation=down  nbits=1  boolean_output=off  mode=Upper Bit Location + Width  bit1=7  base1=LSB of Input  bit0=0  base0=LSB of Input  dbl_ovrd=off  block_type=slice
      settings: infoedit="Extracts a given range of bits from each input sample and presents it at the output.  The output type is ordinarily unsigned with binary point at zero, but can be Boolean when the slice is one bit wide.<P><P>Hardware notes: In hardware this block costs nothing."  block_version=VER_STRING_GOES_HERE
  Slice1 : xbsIndex_r4/Slice  Orientation=down  nbits=1  boolean_output=off  mode=Upper Bit Location + Width  bit1=6  base1=LSB of Input  bit0=0  base0=LSB of Input  dbl_ovrd=off  block_type=slice
      settings: infoedit="Extracts a given range of bits from each input sample and presents it at the output.  The output type is ordinarily unsigned with binary point at zero, but can be Boolean when the slice is one bit wide.<P><P>Hardware notes: In hardware this block costs nothing."  block_version=VER_STRING_GOES_HERE
  Slice2 : xbsIndex_r4/Slice  Orientation=down  nbits=1  boolean_output=off  mode=Upper Bit Location + Width  bit1=8  base1=LSB of Input  bit0=0  base0=LSB of Input  dbl_ovrd=off  block_type=slice
      settings: infoedit="Extracts a given range of bits from each input sample and presents it at the output.  The output type is ordinarily unsigned with binary point at zero, but can be Boolean when the slice is one bit wide.<P><P>Hardware notes: In hardware this block costs nothing."  block_version=VER_STRING_GOES_HERE
  Slice3 : xbsIndex_r4/Slice  Orientation=down  nbits=1  boolean_output=off  mode=Upper Bit Location + Width  bit1=5  base1=LSB of Input  bit0=0  base0=LSB of Input  dbl_ovrd=off  block_type=slice
      settings: infoedit="Extracts a given range of bits from each input sample and presents it at the output.  The output type is ordinarily unsigned with binary point at zero, but can be Boolean when the slice is one bit wide.<P><P>Hardware notes: In hardware this block costs nothing."  block_version=VER_STRING_GOES_HERE
  Slice4 : xbsIndex_r4/Slice  Orientation=down  nbits=1  boolean_output=off  mode=Upper Bit Location + Width  bit1=3  base1=LSB of Input  bit0=0  base0=LSB of Input  dbl_ovrd=off  block_type=slice
      settings: infoedit="Extracts a given range of bits from each input sample and presents it at the output.  The output type is ordinarily unsigned with binary point at zero, but can be Boolean when the slice is one bit wide.<P><P>Hardware notes: In hardware this block costs nothing."  block_version=VER_STRING_GOES_HERE
  Slice5 : xbsIndex_r4/Slice  Orientation=down  nbits=1  boolean_output=off  mode=Upper Bit Location + Width  bit1=2  base1=LSB of Input  bit0=0  base0=LSB of Input  dbl_ovrd=off  block_type=slice
      settings: infoedit="Extracts a given range of bits from each input sample and presents it at the output.  The output type is ordinarily unsigned with binary point at zero, but can be Boolean when the slice is one bit wide.<P><P>Hardware notes: In hardware this block costs nothing."  block_version=VER_STRING_GOES_HERE
  Slice6 : xbsIndex_r4/Slice  Orientation=down  nbits=1  boolean_output=off  mode=Upper Bit Location + Width  bit1=4  base1=LSB of Input  bit0=0  base0=LSB of Input  dbl_ovrd=off  block_type=slice
      settings: infoedit="Extracts a given range of bits from each input sample and presents it at the output.  The output type is ordinarily unsigned with binary point at zero, but can be Boolean when the slice is one bit wide.<P><P>Hardware notes: In hardware this block costs nothing."  block_version=VER_STRING_GOES_HERE
  Slice7 : xbsIndex_r4/Slice  Orientation=down  nbits=1  boolean_output=off  mode=Upper Bit Location + Width  bit1=1  base1=LSB of Input  bit0=0  base0=LSB of Input  dbl_ovrd=off  block_type=slice
      settings: infoedit="Extracts a given range of bits from each input sample and presents it at the output.  The output type is ordinarily unsigned with binary point at zero, but can be Boolean when the slice is one bit wide.<P><P>Hardware notes: In hardware this block costs nothing."  block_version=VER_STRING_GOES_HERE
  Slice8 : xbsIndex_r4/Slice  Orientation=down  nbits=1  boolean_output=off  mode=Upper Bit Location + Width  bit1=0  base1=LSB of Input  bit0=0  base0=LSB of Input  dbl_ovrd=off  block_type=slice
      settings: infoedit="Extracts a given range of bits from each input sample and presents it at the output.  The output type is ordinarily unsigned with binary point at zero, but can be Boolean when the slice is one bit wide.<P><P>Hardware notes: In hardware this block costs nothing."  block_version=VER_STRING_GOES_HERE
  dout : Outport  OutDataType=sfix(16)  OutScaling=2^0
  wires:
  Register1/1 -> Logical2/2, Register2/1
  Slice/1 -> Logical/1
  Slice1/1 -> Logical2/1
  Constant/1 -> Slice/1, Slice1/1, Slice3/1, Slice4/1, Slice5/1, Slice7/1, Slice8/1, Slice6/1, Slice2/1
  Slice2/1 -> Logical3/1
  Logical3/1 -> Logical1/1
  Logical/1 -> Logical1/2
  Slice3/1 -> Logical4/1
  Logical2/1 -> Logical5/1
  Logical4/1 -> Logical5/2
  Logical1/1 -> Logical6/1
  Logical5/1 -> Logical6/2
  Register4/1 -> Register5/1, Logical7/2
  Register6/1 -> Logical11/2, Register7/1
  Register5/1 -> Register6/1, Logical9/2
  Slice4/1 -> Logical7/1
  Slice5/1 -> Logical9/1
  Slice6/1 -> Logical10/1
  Logical10/1 -> Logical8/1
  Logical7/1 -> Logical8/2
  Slice7/1 -> Logical11/1
  Logical9/1 -> Logical12/1
  Logical11/1 -> Logical12/2
  Logical8/1 -> Logical13/1
  Logical12/1 -> Logical13/2
  Register3/1 -> Logical10/2, Register4/1
  Register7/1 -> Logical14/2
  Slice8/1 -> Logical14/1
  Logical6/1 -> Logical15/1
  Logical13/1 -> Logical15/2
  Logical14/1 -> Logical16/2
  Logical15/1 -> Logical16/1
  Register24/1 -> Register0/1, Logical3/2
  Register2/1 -> Register3/1, Logical4/2
  Register0/1 -> Register1/1, Logical/2
  Logical16/1 -> Register10/1
  din/1 -> Register24/1
  rst/1 -> Register0/2, Register3/2, Register6/2, Register7/2, Register5/2, Register4/2, Register2/2, Register1/2, Register24/2, Register10/2
  vin/1 -> Register7/3, Register6/3, Register5/3, Register4/3, Register3/3, Register2/3, Register1/3, Register0/3, Register24/3
  Register10/1 -> dout/1
